simulink model "LeaderFollower"  (R2018a)
settings: Solver=FixedStepAuto  StartTime=0.0  StopTime=300  FixedStep=1  RelTol=1e-3
libraries: simulink x3
settings Model: Creator=wangluo  LastModifiedBy=wangluo

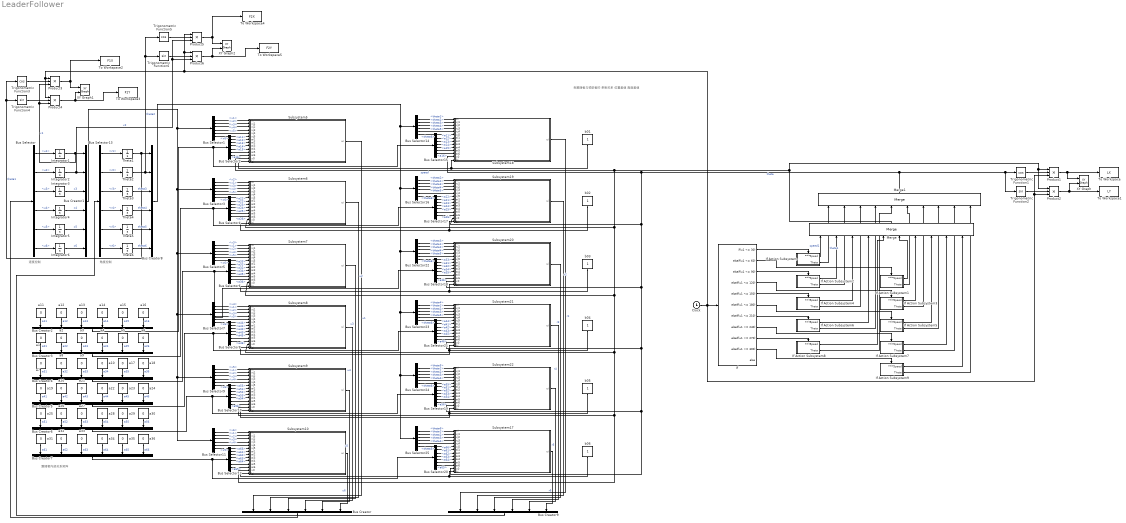
== system LeaderFollower ==
  note: 跟随者内部关系矩阵
  note: 速度控制
  note: 各跟随者与领航者的
      | 牵制关系
      | 位置差值
      | 角度差值
  note: 角度控制
  Bus Creator{,1..9} (10 alike) : BusCreator  Inputs=6
  Bus Selector : BusSelector  OutputSignals=u1,u2,u3,u4,u5,u6
  Bus Selector1 : BusSelector  OutputSignals=x1,x2,x3,x4,x5,x6
  Bus Selector10 : BusSelector  OutputSignals=a55,a51,a52,a53,a54,a56
  Bus Selector11 : BusSelector  OutputSignals=x6,x1,x2,x3,x4,x5
  Bus Selector12 : BusSelector  OutputSignals=a66,a61,a62,a63,a64,a65
  Bus Selector13 : BusSelector  OutputSignals=r1,r2,r3,r4,r5,r6
  Bus Selector14 : BusSelector  OutputSignals=theta1,theta2,theta3,theta4,theta5,theta6
  Bus Selector15 : BusSelector  OutputSignals=a11,a12,a13,a14,a15,a16
  Bus Selector16 : BusSelector  OutputSignals=theta2,theta1,theta3,theta4,theta5,theta6
  Bus Selector17 : BusSelector  OutputSignals=a22,a21,a23,a24,a25,a26
  Bus Selector18 : BusSelector  OutputSignals=a33,a31,a32,a34,a35,a36
  Bus Selector19 : BusSelector  OutputSignals=a55,a51,a52,a53,a54,a56
  Bus Selector2 : BusSelector  OutputSignals=a11,a12,a13,a14,a15,a16
  Bus Selector20 : BusSelector  OutputSignals=a66,a61,a62,a63,a64,a65
  Bus Selector21 : BusSelector  OutputSignals=a44,a41,a42,a43,a45,a46
  Bus Selector22 : BusSelector  OutputSignals=theta3,theta1,theta2,theta4,theta5,theta6
  Bus Selector23 : BusSelector  OutputSignals=theta4,theta1,theta2,theta3,theta5,theta6
  Bus Selector24 : BusSelector  OutputSignals=theta5,theta1,theta2,theta3,theta4,theta6
  Bus Selector25 : BusSelector  OutputSignals=theta6,theta1,theta2,theta3,theta4,theta5
  Bus Selector3 : BusSelector  OutputSignals=x2,x1,x3,x4,x5,x6
  Bus Selector4 : BusSelector  OutputSignals=a22,a21,a23,a24,a25,a26
  Bus Selector5 : BusSelector  OutputSignals=x3,x1,x2,x4,x5,x6
  Bus Selector6 : BusSelector  OutputSignals=a33,a31,a32,a34,a35,a36
  Bus Selector7 : BusSelector  OutputSignals=x4,x1,x2,x3,x5,x6
  Bus Selector8 : BusSelector  OutputSignals=a44,a41,a42,a43,a45,a46
  Bus Selector9 : BusSelector  OutputSignals=x5,x1,x2,x3,x4,x6
  Clock : Clock
      settings: Decimation=280
  If : If  IfExpression=u1 <= 30  ElseIfExpressions=u1 <= 60, u1 <= 90, u1 <= 120, u1 <= 150, u1 <= 180, u1 <= 210, u1 <= 240, u1 <= 270, u1 <= 300
  If Action Subsystem : Subsystem  TreatAsAtomicUnit=on
  If Action Subsystem1 : Subsystem  TreatAsAtomicUnit=on
  If Action Subsystem2 : Subsystem  TreatAsAtomicUnit=on
  If Action Subsystem3 : Subsystem  TreatAsAtomicUnit=on
  If Action Subsystem4 : Subsystem  TreatAsAtomicUnit=on
  If Action Subsystem5 : Subsystem  TreatAsAtomicUnit=on
  If Action Subsystem6 : Subsystem  TreatAsAtomicUnit=on
  If Action Subsystem7 : Subsystem  TreatAsAtomicUnit=on
  If Action Subsystem8 : Subsystem  TreatAsAtomicUnit=on
  If Action Subsystem9 : Subsystem  TreatAsAtomicUnit=on
  Integrator1 : Integrator  InitialCondition=2
  Integrator2 : Integrator  InitialCondition=4
  Integrator3 : Integrator  InitialCondition=6
  Integrator4 : Integrator  InitialCondition=8
  Integrator5 : Integrator  InitialCondition=10
  Integrator6 : Integrator  InitialCondition=2
  Merge : Merge  Inputs=10
  Merge1 : Merge  Inputs=10
  Product{1..6} (6 alike) : Product  Inputs=3
  Subsystem10 : Subsystem
  Subsystem17 : Subsystem
  Subsystem18 : Subsystem
  Subsystem19 : Subsystem
  Subsystem20 : Subsystem
  Subsystem21 : Subsystem
  Subsystem22 : Subsystem
  Subsystem5 : Subsystem
  Subsystem6 : Subsystem
  Subsystem7 : Subsystem
  Subsystem8 : Subsystem
  Subsystem9 : Subsystem
  Theta1 : Integrator
  Theta2 : Integrator  InitialCondition=15
  Theta3 : Integrator  InitialCondition=45
  Theta4 : Integrator  InitialCondition=60
  Theta5 : Integrator  InitialCondition=75
  Theta6 : Integrator  InitialCondition=90
  To Workspace : ToWorkspace  VariableName=LX  SaveFormat=Timeseries  SampleTime=-1
  To Workspace1 : ToWorkspace  VariableName=LY  SaveFormat=Timeseries  SampleTime=-1
  To Workspace2 : ToWorkspace  VariableName=F1X  SaveFormat=Timeseries  SampleTime=-1
  To Workspace3 : ToWorkspace  VariableName=F1Y  SaveFormat=Timeseries  SampleTime=-1
  To Workspace4 : ToWorkspace  VariableName=F2X  SaveFormat=Timeseries  SampleTime=-1
  To Workspace5 : ToWorkspace  VariableName=F2Y  SaveFormat=Timeseries  SampleTime=-1
  Trigonometric Function1 : Trigonometry  Operator=cos
  Trigonometric Function2 : Trigonometry
  Trigonometric Function3 : Trigonometry  Operator=cos
  Trigonometric Function4 : Trigonometry
  Trigonometric Function5 : Trigonometry  Operator=cos
  Trigonometric Function6 : Trigonometry
  XY Graph : simulink/Sinks/XY Graph  xmin=-10  xmax=500  ymin=-10  ymax=500  st=-1
  XY Graph1 : simulink/Sinks/XY Graph  xmin=-10  xmax=500  ymin=-10  ymax=500  st=-1
  XY Graph2 : simulink/Sinks/XY Graph  xmin=-10  xmax=500  ymin=-10  ymax=500  st=-1
  a{1..36} (36 alike) : Constant  Value=0
  b01 : Constant
  b02 : Constant
  b03 : Constant
  b04 : Constant
  b05 : Constant
  b06 : Constant
  wires:
  a8/1 -> Bus Creator4/2  "a32"
  a35/1 -> Bus Creator7/5  "a65"
  Integrator1/1 -> Product4/3, Product3/3, Bus Creator1/1  "x1"
  a19/1 -> Bus Creator5/1  "a41"
  Bus Selector12/1 -> Subsystem10/7(ai1)  "<a66>"
  Bus Selector6/3 -> Subsystem7/9(ai3)  "<a32>"
  Bus Selector9/6 -> Subsystem9/6(xj5)  "<x6>"
  a26/1 -> Bus Creator6/2  "a52"
  Bus Selector4/2 -> Subsystem6/8(ai2)  "<a21>"
  Bus Selector8/1 -> Subsystem8/7(ai1)  "<a44>"
  Integrator3/1 -> Bus Creator1/3  "x3"
  Subsystem8/1(ui) -> Bus Creator/4  "u4"
  Bus Selector10/2 -> Subsystem9/8(ai2)  "<a51>"
  Bus Selector2/4 -> Subsystem5/10(ai4)  "<a14>"
  Bus Selector8/3 -> Subsystem8/9(ai3)  "<a42>"
  Bus Selector12/5 -> Subsystem10/11(ai5)  "<a64>"
  Bus Selector3/5 -> Subsystem6/5(xj4)  "<x5>"
  Bus Selector8/2 -> Subsystem8/8(ai2)  "<a41>"
  a29/1 -> Bus Creator6/5  "a55"
  Bus Selector4/6 -> Subsystem6/12(ai6)  "<a26>"
  Integrator6/1 -> Bus Creator1/6  "x6"
  a23/1 -> Bus Creator5/5  "a45"
  a34/1 -> Bus Creator7/4  "a64"
  Bus Selector3/2 -> Subsystem6/2(xj1)  "<x1>"
  a16/1 -> Bus Creator2/6  "a16"
  a2/1 -> Bus Creator3/2  "a22"
  Bus Selector6/6 -> Subsystem7/12(ai6)  "<a36>"
  Bus Creator4/1 -> Bus Selector18/1, Bus Selector6/1
  Bus Selector2/2 -> Subsystem5/8(ai2)  "<a12>"
  a22/1 -> Bus Creator5/4  "a44"
  Bus Selector7/1 -> Subsystem8/1(xi)  "<x4>"
  Bus Selector7/5 -> Subsystem8/5(xj4)  "<x5>"
  Bus Selector7/2 -> Subsystem8/2(xj1)  "<x1>"
  Bus Creator1/1 -> Bus Selector11/1, Bus Selector9/1, Bus Selector7/1, Bus Selector5/1, Bus Selector3/1, Bus Selector1/1
  Bus Selector1/3 -> Subsystem5/3(xj2)  "<x3>"
  Bus Selector9/3 -> Subsystem9/3(xj2)  "<x2>"
  Bus Selector3/3 -> Subsystem6/3(xj2)  "<x3>"
  a27/1 -> Bus Creator6/3  "a53"
  a31/1 -> Bus Creator7/1  "a61"
  Bus Selector2/5 -> Subsystem5/11(ai5)  "<a15>"
  a15/1 -> Bus Creator2/5  "a15"
  a17/1 -> Bus Creator4/5  "a35"
  Bus Selector9/2 -> Subsystem9/2(xj1)  "<x1>"
  a1/1 -> Bus Creator3/1  "a21"
  Bus Selector12/6 -> Subsystem10/12(ai6)  "<a65>"
  a18/1 -> Bus Creator4/6  "a36"
  a5/1 -> Bus Creator3/5  "a25"
  Bus Selector2/1 -> Subsystem5/7(ai1)  "<a11>"
  Bus Selector4/1 -> Subsystem6/7(ai1)  "<a22>"
  Bus Selector11/4 -> Subsystem10/4(xj3)  "<x3>"
  Bus Selector7/4 -> Subsystem8/4(xj3)  "<x3>"
  Bus Selector12/2 -> Subsystem10/8(ai2)  "<a61>"
  Bus Selector7/3 -> Subsystem8/3(xj2)  "<x2>"
  Bus Selector11/3 -> Subsystem10/3(xj2)  "<x2>"
  a11/1 -> Bus Creator2/1  "a11"
  Bus Creator/1 -> Bus Selector/1
  Bus Selector5/2 -> Subsystem7/2(xj1)  "<x1>"
  Bus Selector2/6 -> Subsystem5/12(ai6)  "<a16>"
  a25/1 -> Bus Creator6/1  "a51"
  Bus Selector1/6 -> Subsystem5/6(xj5)  "<x6>"
  Bus Selector5/6 -> Subsystem7/6(xj5)  "<x6>"
  Bus Selector8/6 -> Subsystem8/12(ai6)  "<a46>"
  Bus Creator7/1 -> Bus Selector20/1, Bus Selector12/1
  Bus Selector5/5 -> Subsystem7/5(xj4)  "<x5>"
  Bus Selector3/1 -> Subsystem6/1(xi)  "<x2>"
  Bus Selector6/4 -> Subsystem7/10(ai4)  "<a34>"
  Bus Selector5/4 -> Subsystem7/4(xj3)  "<x4>"
  a28/1 -> Bus Creator6/4  "a54"
  Bus Selector2/3 -> Subsystem5/9(ai3)  "<a13>"
  Subsystem6/1(ui) -> Bus Creator/2  "u2"
  a13/1 -> Bus Creator2/3  "a13"
  a32/1 -> Bus Creator7/2  "a62"
  Bus Selector1/4 -> Subsystem5/4(xj3)  "<x4>"
  Subsystem5/1(ui) -> Bus Creator/1  "u1"
  Bus Selector10/3 -> Subsystem9/9(ai3)  "<a52>"
  Integrator4/1 -> Bus Creator1/4  "x4"
  Bus Selector5/3 -> Subsystem7/3(xj2)  "<x2>"
  Bus Selector6/2 -> Subsystem7/8(ai2)  "<a31>"
  Bus Selector4/4 -> Subsystem6/10(ai4)  "<a24>"
  Bus Selector11/6 -> Subsystem10/6(xj5)  "<x5>"
  a36/1 -> Bus Creator7/6  "a66"
  Bus Selector4/5 -> Subsystem6/11(ai5)  "<a25>"
  Bus Selector4/3 -> Subsystem6/9(ai3)  "<a23>"
  Bus Selector3/6 -> Subsystem6/6(xj5)  "<x6>"
  Bus Selector5/1 -> Subsystem7/1(xi)  "<x3>"
  Bus Creator6/1 -> Bus Selector19/1, Bus Selector10/1
  Bus Selector7/6 -> Subsystem8/6(xj5)  "<x6>"
  Bus Selector12/4 -> Subsystem10/10(ai4)  "<a63>"
  Bus Selector8/4 -> Subsystem8/10(ai4)  "<a43>"
  Integrator5/1 -> Bus Creator1/5  "x5"
  Bus Selector10/5 -> Subsystem9/11(ai5)  "<a54>"
  Bus Selector1/1 -> Subsystem5/1(xi)  "<x1>"
  Integrator2/1 -> Product6/3, Product5/3, Bus Creator1/2  "x2"
  Bus Selector10/4 -> Subsystem9/10(ai4)  "<a53>"
  Bus Selector8/5 -> Subsystem8/11(ai5)  "<a45>"
  Bus Selector9/1 -> Subsystem9/1(xi)  "<x5>"
  Bus Selector6/1 -> Subsystem7/7(ai1)  "<a33>"
  a33/1 -> Bus Creator7/3  "a63"
  Bus Selector9/4 -> Subsystem9/4(xj3)  "<x3>"
  Subsystem10/1(ui) -> Bus Creator/6  "u6"
  Bus Selector3/4 -> Subsystem6/4(xj3)  "<x4>"
  Bus Creator2/1 -> Bus Selector2/1, Bus Selector15/1
  a21/1 -> Bus Creator5/3  "a43"
  a12/1 -> Bus Creator2/2  "a12"
  a24/1 -> Bus Creator5/6  "a46"
  Bus Selector11/2 -> Subsystem10/2(xj1)  "<x1>"
  Bus Selector6/5 -> Subsystem7/11(ai5)  "<a35>"
  Bus Selector10/6 -> Subsystem9/12(ai6)  "<a56>"
  Bus Selector11/5 -> Subsystem10/5(xj4)  "<x4>"
  Bus Selector9/5 -> Subsystem9/5(xj4)  "<x4>"
  Subsystem7/1(ui) -> Bus Creator/3  "u3"
  a3/1 -> Bus Creator3/3  "a23"
  Bus Selector11/1 -> Subsystem10/1(xi)  "<x6>"
  a20/1 -> Bus Creator5/2  "a42"
  Bus Selector10/1 -> Subsystem9/7(ai1)  "<a55>"
  a6/1 -> Bus Creator3/6  "a26"
  Bus Selector1/5 -> Subsystem5/5(xj4)  "<x5>"
  Bus Selector12/3 -> Subsystem10/9(ai3)  "<a62>"
  a4/1 -> Bus Creator3/4  "a24"
  a10/1 -> Bus Creator4/4  "a34"
  Bus Creator3/1 -> Bus Selector4/1, Bus Selector17/1
  a7/1 -> Bus Creator4/1  "a31"
  Bus Creator5/1 -> Bus Selector8/1, Bus Selector21/1
  a30/1 -> Bus Creator6/6  "a56"
  Bus Selector1/2 -> Subsystem5/2(xj1)  "<x2>"
  a9/1 -> Bus Creator4/3  "a33"
  Subsystem9/1(ui) -> Bus Creator/5  "u5"
  a14/1 -> Bus Creator2/4  "a14"
  Bus Selector/1 -> Integrator1/1  "<u1>"
  Bus Selector/2 -> Integrator2/1  "<u2>"
  Bus Selector/3 -> Integrator3/1  "<u3>"
  Bus Selector/4 -> Integrator4/1  "<u4>"
  Bus Selector/5 -> Integrator5/1  "<u5>"
  Bus Selector/6 -> Integrator6/1  "<u6>"
  Theta1/1 -> Trigonometric Function3/1, Trigonometric Function4/1, Bus Creator8/1  "theta1"
  Theta2/1 -> Trigonometric Function5/1, Trigonometric Function6/1, Bus Creator8/2  "theta2"
  Theta3/1 -> Bus Creator8/3  "theta3"
  Theta5/1 -> Bus Creator8/5  "theta5"
  Theta6/1 -> Bus Creator8/6  "theta6"
  Theta4/1 -> Bus Creator8/4  "theta4"
  Bus Selector13/1 -> Theta1/1  "<r1>"
  Bus Selector13/2 -> Theta2/1  "<r2>"
  Bus Selector13/3 -> Theta3/1  "<r3>"
  Bus Selector13/4 -> Theta4/1  "<r4>"
  Bus Selector13/5 -> Theta5/1  "<r5>"
  Bus Selector13/6 -> Theta6/1  "<r6>"
  Bus Selector14/1 -> Subsystem18/1(xi)  "<theta1>"
  Bus Selector14/2 -> Subsystem18/2(xj1)  "<theta2>"
  Bus Selector14/3 -> Subsystem18/3(xj2)  "<theta3>"
  Bus Selector14/4 -> Subsystem18/4(xj3)  "<theta4>"
  Bus Selector14/5 -> Subsystem18/5(xj4)  "<theta5>"
  Bus Selector14/6 -> Subsystem18/6(xj5)  "<theta6>"
  Bus Creator8/1 -> Bus Selector23/1, Bus Selector25/1, Bus Selector24/1, Bus Selector22/1, Bus Selector16/1, Bus Selector14/1
  Subsystem17/1(ui) -> Bus Creator9/6  "r6"
  Bus Selector15/1 -> Subsystem18/7(ai1)  "<a11>"
  Bus Selector15/2 -> Subsystem18/8(ai2)  "<a12>"
  Bus Selector15/3 -> Subsystem18/9(ai3)  "<a13>"
  Bus Selector15/4 -> Subsystem18/10(ai4)  "<a14>"
  Bus Selector15/5 -> Subsystem18/11(ai5)  "<a15>"
  Bus Selector15/6 -> Subsystem18/12(ai6)  "<a16>"
  Bus Selector17/1 -> Subsystem19/7(ai1)  "<a22>"
  Bus Selector17/2 -> Subsystem19/8(ai2)  "<a21>"
  Bus Selector17/3 -> Subsystem19/9(ai3)  "<a23>"
  Bus Selector17/4 -> Subsystem19/10(ai4)  "<a24>"
  Bus Selector17/5 -> Subsystem19/11(ai5)  "<a25>"
  Bus Selector17/6 -> Subsystem19/12(ai6)  "<a26>"
  Bus Selector16/1 -> Subsystem19/1(xi)  "<theta2>"
  Bus Selector16/2 -> Subsystem19/2(xj1)  "<theta1>"
  Bus Selector16/3 -> Subsystem19/3(xj2)  "<theta3>"
  Bus Selector16/4 -> Subsystem19/4(xj3)  "<theta4>"
  Bus Selector16/5 -> Subsystem19/5(xj4)  "<theta5>"
  Bus Selector16/6 -> Subsystem19/6(xj5)  "<theta6>"
  Bus Selector18/1 -> Subsystem20/7(ai1)  "<a33>"
  Bus Selector18/2 -> Subsystem20/8(ai2)  "<a31>"
  Bus Selector18/3 -> Subsystem20/9(ai3)  "<a32>"
  Bus Selector18/4 -> Subsystem20/10(ai4)  "<a34>"
  Bus Selector18/5 -> Subsystem20/11(ai5)  "<a35>"
  Bus Selector18/6 -> Subsystem20/12(ai6)  "<a36>"
  Bus Selector21/1 -> Subsystem21/7(ai1)  "<a44>"
  Bus Selector21/2 -> Subsystem21/8(ai2)  "<a41>"
  Bus Selector21/3 -> Subsystem21/9(ai3)  "<a42>"
  Bus Selector21/4 -> Subsystem21/10(ai4)  "<a43>"
  Bus Selector21/5 -> Subsystem21/11(ai5)  "<a45>"
  Bus Selector21/6 -> Subsystem21/12(ai6)  "<a46>"
  Bus Selector19/1 -> Subsystem22/7(ai1)  "<a55>"
  Bus Selector19/2 -> Subsystem22/8(ai2)  "<a51>"
  Bus Selector19/3 -> Subsystem22/9(ai3)  "<a52>"
  Bus Selector19/4 -> Subsystem22/10(ai4)  "<a53>"
  Bus Selector19/5 -> Subsystem22/11(ai5)  "<a54>"
  Bus Selector19/6 -> Subsystem22/12(ai6)  "<a56>"
  Bus Selector20/1 -> Subsystem17/7(ai1)  "<a66>"
  Bus Selector20/2 -> Subsystem17/8(ai2)  "<a61>"
  Bus Selector20/3 -> Subsystem17/9(ai3)  "<a62>"
  Bus Selector20/4 -> Subsystem17/10(ai4)  "<a63>"
  Bus Selector20/5 -> Subsystem17/11(ai5)  "<a64>"
  Bus Selector20/6 -> Subsystem17/12(ai6)  "<a65>"
  Subsystem22/1(ui) -> Bus Creator9/5  "r5"
  Subsystem21/1(ui) -> Bus Creator9/4  "r4"
  Subsystem20/1(ui) -> Bus Creator9/3  "r3"
  Subsystem18/1(ui) -> Bus Creator9/1  "r1"
  Subsystem19/1(ui) -> Bus Creator9/2  "r2"
  Bus Creator9/1 -> Bus Selector13/1
  Bus Selector22/1 -> Subsystem20/1(xi)  "<theta3>"
  Bus Selector22/2 -> Subsystem20/2(xj1)  "<theta1>"
  Bus Selector22/3 -> Subsystem20/3(xj2)  "<theta2>"
  Bus Selector22/4 -> Subsystem20/4(xj3)  "<theta4>"
  Bus Selector22/5 -> Subsystem20/5(xj4)  "<theta5>"
  Bus Selector22/6 -> Subsystem20/6(xj5)  "<theta6>"
  Bus Selector23/1 -> Subsystem21/1(xi)  "<theta4>"
  Bus Selector23/2 -> Subsystem21/2(xj1)  "<theta1>"
  Bus Selector23/3 -> Subsystem21/3(xj2)  "<theta2>"
  Bus Selector23/4 -> Subsystem21/4(xj3)  "<theta3>"
  Bus Selector23/5 -> Subsystem21/5(xj4)  "<theta5>"
  Bus Selector23/6 -> Subsystem21/6(xj5)  "<theta6>"
  Bus Selector25/1 -> Subsystem17/1(xi)  "<theta6>"
  Bus Selector25/2 -> Subsystem17/2(xj1)  "<theta1>"
  Bus Selector25/3 -> Subsystem17/3(xj2)  "<theta2>"
  Bus Selector25/4 -> Subsystem17/4(xj3)  "<theta3>"
  Bus Selector25/5 -> Subsystem17/5(xj4)  "<theta4>"
  Bus Selector25/6 -> Subsystem17/6(xj5)  "<theta5>"
  Bus Selector24/1 -> Subsystem22/1(xi)  "<theta5>"
  Bus Selector24/2 -> Subsystem22/2(xj1)  "<theta1>"
  Bus Selector24/3 -> Subsystem22/3(xj2)  "<theta2>"
  Bus Selector24/4 -> Subsystem22/4(xj3)  "<theta3>"
  Bus Selector24/5 -> Subsystem22/5(xj4)  "<theta4>"
  Bus Selector24/6 -> Subsystem22/6(xj5)  "<theta6>"
  b01/1 -> Subsystem18/14(bi), Subsystem5/14(bi)
  b02/1 -> Subsystem19/14(bi), Subsystem6/14(bi)
  b03/1 -> Subsystem20/14(bi), Subsystem7/14(bi)
  b04/1 -> Subsystem8/14(bi), Subsystem21/14(bi)
  b05/1 -> Subsystem9/14(bi), Subsystem22/14(bi)
  b06/1 -> Subsystem17/14(bi), Subsystem10/14(bi)
  Merge1/1 -> Subsystem17/13(x0), Subsystem22/13(x0), Subsystem21/13(x0), Subsystem20/13(x0), Subsystem19/13(x0), Subsystem18/13(x0), Trigonometric Function2/1, Trigonometric Function1/1  "theta"
  Clock/1 -> Product5/1, Product6/1, Product4/1, Product3/1, Product1/3, Product2/3, If/1
  Merge/1 -> Product1/1, Product2/1, Subsystem10/13(x0), Subsystem9/13(x0), Subsystem8/13(x0), Subsystem7/13(x0), Subsystem6/13(x0), Subsystem5/13(x0)  "speed"
  If/1 -> If Action Subsystem/Action
  If/3 -> If Action Subsystem2/Action
  If/5 -> If Action Subsystem4/Action
  If/7 -> If Action Subsystem6/Action
  If/9 -> If Action Subsystem8/Action
  If/2 -> If Action Subsystem1/Action
  If/10 -> If Action Subsystem9/Action
  If/8 -> If Action Subsystem7/Action
  If/6 -> If Action Subsystem5/Action
  If/4 -> If Action Subsystem3/Action
  If Action Subsystem/1(Speed) -> Merge/1  "speed1"
  If Action Subsystem2/1(Speed) -> Merge/2
  If Action Subsystem4/1(Speed) -> Merge/3
  If Action Subsystem6/1(Speed) -> Merge/4
  If Action Subsystem8/1(Speed) -> Merge/5
  If Action Subsystem1/1(Speed) -> Merge/6
  If Action Subsystem3/1(Speed) -> Merge/7
  If Action Subsystem9/1(Speed) -> Merge/10
  If Action Subsystem7/1(Speed) -> Merge/9
  If Action Subsystem5/1(Speed) -> Merge/8
  If Action Subsystem/2(Theta) -> Merge1/1  "theta1"
  If Action Subsystem2/2(Theta) -> Merge1/2
  If Action Subsystem4/2(Theta) -> Merge1/3
  If Action Subsystem6/2(Theta) -> Merge1/4
  If Action Subsystem8/2(Theta) -> Merge1/5
  If Action Subsystem1/2(Theta) -> Merge1/6
  If Action Subsystem3/2(Theta) -> Merge1/7
  If Action Subsystem5/2(Theta) -> Merge1/8
  If Action Subsystem7/2(Theta) -> Merge1/9
  If Action Subsystem9/2(Theta) -> Merge1/10
  Trigonometric Function1/1 -> Product1/2
  Trigonometric Function2/1 -> Product2/2
  Product1/1 -> To Workspace/1, XY Graph/1
  Product2/1 -> To Workspace1/1, XY Graph/2
  Product3/1 -> To Workspace2/1, XY Graph1/1
  Product4/1 -> To Workspace3/1, XY Graph1/2
  Trigonometric Function3/1 -> Product3/2
  Trigonometric Function4/1 -> Product4/2
  Product5/1 -> To Workspace4/1, XY Graph2/1
  Product6/1 -> To Workspace5/1, XY Graph2/2
  Trigonometric Function5/1 -> Product5/2
  Trigonometric Function6/1 -> Product6/2

== system LeaderFollower/If Action Subsystem ==
  Action Port : ActionPort  ActionType=then
  b1 : Constant  Value=5
  b2 : Constant  Value=pi/180*90
  Speed : Outport
  Theta : Outport  Port=2
  wires:
  b1/1 -> Speed/1
  b2/1 -> Theta/1

== system LeaderFollower/If Action Subsystem1 ==
  Action Port : ActionPort  ActionType=elseif
  b1 : Constant  Value=5
  b2 : Constant  Value=pi/180*0
  Speed : Outport
  Theta : Outport  Port=2
  wires:
  b1/1 -> Speed/1
  b2/1 -> Theta/1

== system LeaderFollower/If Action Subsystem2 ==
  Action Port : ActionPort  ActionType=elseif
  b1 : Constant  Value=5
  b2 : Constant  Value=pi/180*45
  Speed : Outport
  Theta : Outport  Port=2
  wires:
  b1/1 -> Speed/1
  b2/1 -> Theta/1

== system LeaderFollower/If Action Subsystem3 ==
  Action Port : ActionPort  ActionType=elseif
  b1 : Constant  Value=5
  b2 : Constant  Value=pi/180*90
  Speed : Outport
  Theta : Outport  Port=2
  wires:
  b1/1 -> Speed/1
  b2/1 -> Theta/1

== system LeaderFollower/If Action Subsystem4 ==
  Action Port : ActionPort  ActionType=elseif
  b1 : Constant  Value=5
  b2 : Constant  Value=pi/180*45
  Speed : Outport
  Theta : Outport  Port=2
  wires:
  b1/1 -> Speed/1
  b2/1 -> Theta/1

== system LeaderFollower/If Action Subsystem5 ==
  Action Port : ActionPort  ActionType=elseif
  b1 : Constant  Value=5
  b2 : Constant  Value=pi/180*0
  Speed : Outport
  Theta : Outport  Port=2
  wires:
  b1/1 -> Speed/1
  b2/1 -> Theta/1

== system LeaderFollower/If Action Subsystem6 ==
  Action Port : ActionPort  ActionType=elseif
  b1 : Constant  Value=5
  b2 : Constant  Value=pi/180*(-45)
  Speed : Outport
  Theta : Outport  Port=2
  wires:
  b1/1 -> Speed/1
  b2/1 -> Theta/1

== system LeaderFollower/If Action Subsystem7 ==
  Action Port : ActionPort  ActionType=elseif
  b1 : Constant  Value=5
  b2 : Constant  Value=pi/180*(-90)
  Speed : Outport
  Theta : Outport  Port=2
  wires:
  b1/1 -> Speed/1
  b2/1 -> Theta/1

== system LeaderFollower/If Action Subsystem8 ==
  Action Port : ActionPort  ActionType=elseif
  b1 : Constant  Value=5
  b2 : Constant  Value=pi/180*(-45)
  Speed : Outport
  Theta : Outport  Port=2
  wires:
  b1/1 -> Speed/1
  b2/1 -> Theta/1

== system LeaderFollower/If Action Subsystem9 ==
  Action Port : ActionPort  ActionType=elseif
  b1 : Constant  Value=5
  b2 : Constant  Value=pi/180*0
  Speed : Outport
  Theta : Outport  Port=2
  wires:
  b1/1 -> Speed/1
  b2/1 -> Theta/1

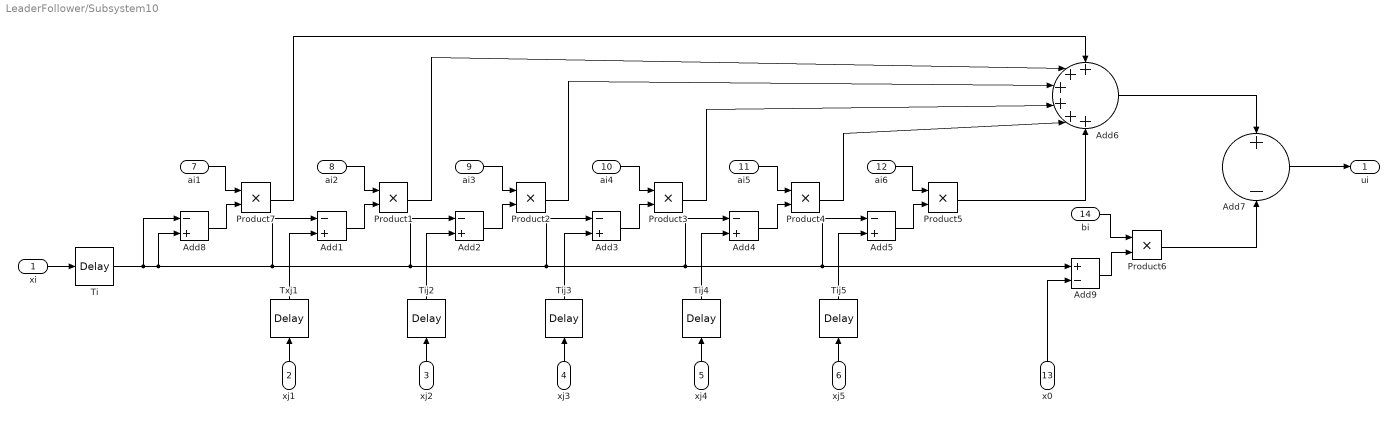
== system LeaderFollower/Subsystem10 ==
  xi : Inport
  xj1 : Inport  Port=2
  xj2 : Inport  Port=3
  xj3 : Inport  Port=4
  xj4 : Inport  Port=5
  xj5 : Inport  Port=6
  ai1 : Inport  Port=7
  ai2 : Inport  Port=8
  ai3 : Inport  Port=9
  ai4 : Inport  Port=10
  ai5 : Inport  Port=11
  ai6 : Inport  Port=12
  x0 : Inport  Port=13
  bi : Inport  Port=14
  Add{1..5,8} (6 alike) : Sum  Inputs=-+
  Add6 : Sum  Inputs=++++++
  Add7 : Sum  Inputs=+-
  Add9 : Sum  Inputs=+-
  Product{1..7} (7 alike) : Product
  Ti : TransportDelay  DelayTime=0
  Tij{2..5} (4 alike) : TransportDelay  DelayTime=0
  Txj1 : TransportDelay  DelayTime=0
  ui : Outport
  wires:
  Product7/1 -> Add6/1
  Add8/1 -> Product7/2
  ai1/1 -> Product7/1
  ai2/1 -> Product1/1
  Add1/1 -> Product1/2
  ai3/1 -> Product2/1
  Add2/1 -> Product2/2
  ai4/1 -> Product3/1
  Add3/1 -> Product3/2
  ai5/1 -> Product4/1
  Add4/1 -> Product4/2
  ai6/1 -> Product5/1
  Add5/1 -> Product5/2
  xi/1 -> Ti/1
  xj5/1 -> Tij5/1
  xj1/1 -> Txj1/1
  Ti/1 -> Add5/1, Add9/1, Add4/1, Add3/1, Add2/1, Add1/1, Add8/2, Add8/1
  Txj1/1 -> Add1/2
  xj2/1 -> Tij2/1
  xj3/1 -> Tij3/1
  xj4/1 -> Tij4/1
  Tij5/1 -> Add5/2
  Tij2/1 -> Add2/2
  Tij3/1 -> Add3/2
  Tij4/1 -> Add4/2
  Product5/1 -> Add6/6
  Product4/1 -> Add6/5
  Product3/1 -> Add6/4
  Product2/1 -> Add6/3
  Product1/1 -> Add6/2
  Add9/1 -> Product6/2
  bi/1 -> Product6/1
  x0/1 -> Add9/2
  Add6/1 -> Add7/1
  Product6/1 -> Add7/2
  Add7/1 -> ui/1

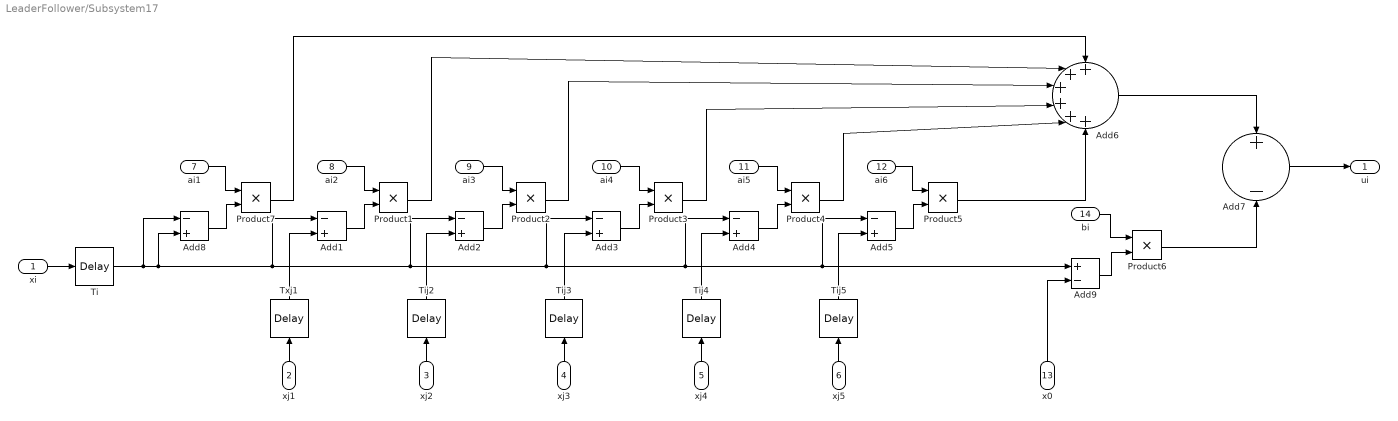
== system LeaderFollower/Subsystem17 ==
  xi : Inport
  xj1 : Inport  Port=2
  xj2 : Inport  Port=3
  xj3 : Inport  Port=4
  xj4 : Inport  Port=5
  xj5 : Inport  Port=6
  ai1 : Inport  Port=7
  ai2 : Inport  Port=8
  ai3 : Inport  Port=9
  ai4 : Inport  Port=10
  ai5 : Inport  Port=11
  ai6 : Inport  Port=12
  x0 : Inport  Port=13
  bi : Inport  Port=14
  Add{1..5,8} (6 alike) : Sum  Inputs=-+
  Add6 : Sum  Inputs=++++++
  Add7 : Sum  Inputs=+-
  Add9 : Sum  Inputs=+-
  Product{1..7} (7 alike) : Product
  Ti : TransportDelay  DelayTime=0
  Tij{2..5} (4 alike) : TransportDelay  DelayTime=0
  Txj1 : TransportDelay  DelayTime=0
  ui : Outport
  wires:
  Product7/1 -> Add6/1
  Add8/1 -> Product7/2
  ai1/1 -> Product7/1
  ai2/1 -> Product1/1
  Add1/1 -> Product1/2
  ai3/1 -> Product2/1
  Add2/1 -> Product2/2
  ai4/1 -> Product3/1
  Add3/1 -> Product3/2
  ai5/1 -> Product4/1
  Add4/1 -> Product4/2
  ai6/1 -> Product5/1
  Add5/1 -> Product5/2
  xi/1 -> Ti/1
  xj5/1 -> Tij5/1
  xj1/1 -> Txj1/1
  Ti/1 -> Add5/1, Add9/1, Add4/1, Add3/1, Add2/1, Add1/1, Add8/2, Add8/1
  Txj1/1 -> Add1/2
  xj2/1 -> Tij2/1
  xj3/1 -> Tij3/1
  xj4/1 -> Tij4/1
  Tij5/1 -> Add5/2
  Tij2/1 -> Add2/2
  Tij3/1 -> Add3/2
  Tij4/1 -> Add4/2
  Product5/1 -> Add6/6
  Product4/1 -> Add6/5
  Product3/1 -> Add6/4
  Product2/1 -> Add6/3
  Product1/1 -> Add6/2
  Add9/1 -> Product6/2
  bi/1 -> Product6/1
  x0/1 -> Add9/2
  Add6/1 -> Add7/1
  Product6/1 -> Add7/2
  Add7/1 -> ui/1

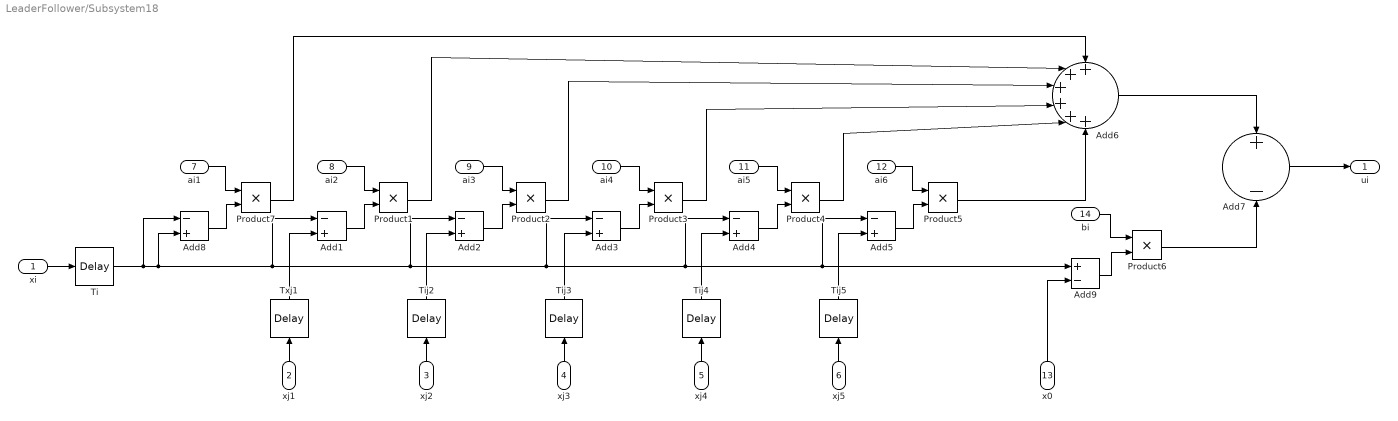
== system LeaderFollower/Subsystem18 ==
  xi : Inport
  xj1 : Inport  Port=2
  xj2 : Inport  Port=3
  xj3 : Inport  Port=4
  xj4 : Inport  Port=5
  xj5 : Inport  Port=6
  ai1 : Inport  Port=7
  ai2 : Inport  Port=8
  ai3 : Inport  Port=9
  ai4 : Inport  Port=10
  ai5 : Inport  Port=11
  ai6 : Inport  Port=12
  x0 : Inport  Port=13
  bi : Inport  Port=14
  Add{1..5,8} (6 alike) : Sum  Inputs=-+
  Add6 : Sum  Inputs=++++++
  Add7 : Sum  Inputs=+-
  Add9 : Sum  Inputs=+-
  Product{1..7} (7 alike) : Product
  Ti : TransportDelay  DelayTime=0
  Tij{2..5} (4 alike) : TransportDelay  DelayTime=0
  Txj1 : TransportDelay  DelayTime=0
  ui : Outport
  wires:
  Product7/1 -> Add6/1
  Add8/1 -> Product7/2
  ai1/1 -> Product7/1
  ai2/1 -> Product1/1
  Add1/1 -> Product1/2
  ai3/1 -> Product2/1
  Add2/1 -> Product2/2
  ai4/1 -> Product3/1
  Add3/1 -> Product3/2
  ai5/1 -> Product4/1
  Add4/1 -> Product4/2
  ai6/1 -> Product5/1
  Add5/1 -> Product5/2
  xi/1 -> Ti/1
  xj5/1 -> Tij5/1
  xj1/1 -> Txj1/1
  Ti/1 -> Add5/1, Add9/1, Add4/1, Add3/1, Add2/1, Add1/1, Add8/2, Add8/1
  Txj1/1 -> Add1/2
  xj2/1 -> Tij2/1
  xj3/1 -> Tij3/1
  xj4/1 -> Tij4/1
  Tij5/1 -> Add5/2
  Tij2/1 -> Add2/2
  Tij3/1 -> Add3/2
  Tij4/1 -> Add4/2
  Product5/1 -> Add6/6
  Product4/1 -> Add6/5
  Product3/1 -> Add6/4
  Product2/1 -> Add6/3
  Product1/1 -> Add6/2
  Add9/1 -> Product6/2
  bi/1 -> Product6/1
  x0/1 -> Add9/2
  Add6/1 -> Add7/1
  Product6/1 -> Add7/2
  Add7/1 -> ui/1

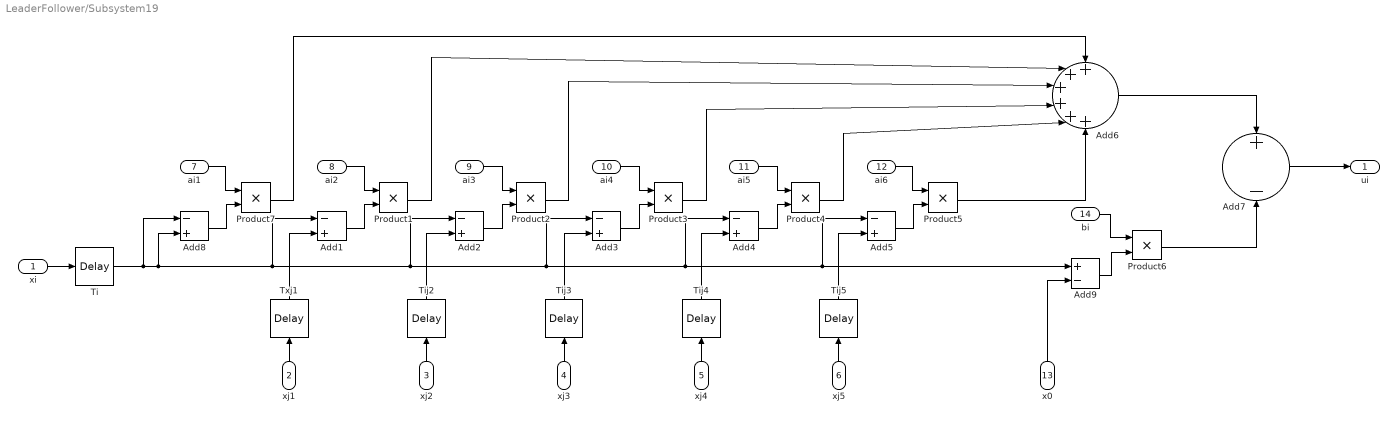
== system LeaderFollower/Subsystem19 ==
  xi : Inport
  xj1 : Inport  Port=2
  xj2 : Inport  Port=3
  xj3 : Inport  Port=4
  xj4 : Inport  Port=5
  xj5 : Inport  Port=6
  ai1 : Inport  Port=7
  ai2 : Inport  Port=8
  ai3 : Inport  Port=9
  ai4 : Inport  Port=10
  ai5 : Inport  Port=11
  ai6 : Inport  Port=12
  x0 : Inport  Port=13
  bi : Inport  Port=14
  Add{1..5,8} (6 alike) : Sum  Inputs=-+
  Add6 : Sum  Inputs=++++++
  Add7 : Sum  Inputs=+-
  Add9 : Sum  Inputs=+-
  Product{1..7} (7 alike) : Product
  Ti : TransportDelay  DelayTime=0
  Tij{2..5} (4 alike) : TransportDelay  DelayTime=0
  Txj1 : TransportDelay  DelayTime=0
  ui : Outport
  wires:
  Product7/1 -> Add6/1
  Add8/1 -> Product7/2
  ai1/1 -> Product7/1
  ai2/1 -> Product1/1
  Add1/1 -> Product1/2
  ai3/1 -> Product2/1
  Add2/1 -> Product2/2
  ai4/1 -> Product3/1
  Add3/1 -> Product3/2
  ai5/1 -> Product4/1
  Add4/1 -> Product4/2
  ai6/1 -> Product5/1
  Add5/1 -> Product5/2
  xi/1 -> Ti/1
  xj5/1 -> Tij5/1
  xj1/1 -> Txj1/1
  Ti/1 -> Add5/1, Add9/1, Add4/1, Add3/1, Add2/1, Add1/1, Add8/2, Add8/1
  Txj1/1 -> Add1/2
  xj2/1 -> Tij2/1
  xj3/1 -> Tij3/1
  xj4/1 -> Tij4/1
  Tij5/1 -> Add5/2
  Tij2/1 -> Add2/2
  Tij3/1 -> Add3/2
  Tij4/1 -> Add4/2
  Product5/1 -> Add6/6
  Product4/1 -> Add6/5
  Product3/1 -> Add6/4
  Product2/1 -> Add6/3
  Product1/1 -> Add6/2
  Add9/1 -> Product6/2
  bi/1 -> Product6/1
  x0/1 -> Add9/2
  Add6/1 -> Add7/1
  Product6/1 -> Add7/2
  Add7/1 -> ui/1

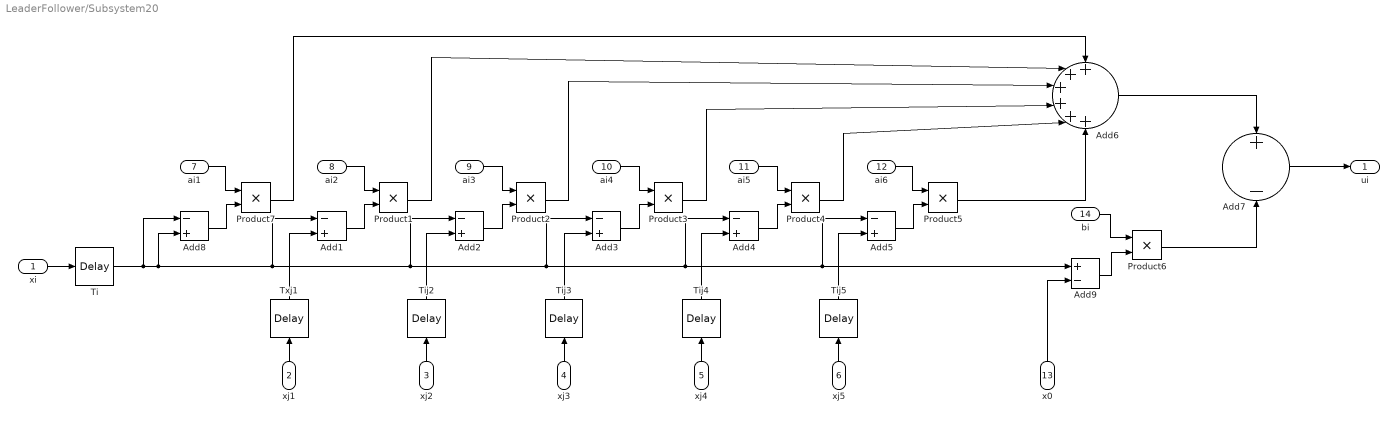
== system LeaderFollower/Subsystem20 ==
  xi : Inport
  xj1 : Inport  Port=2
  xj2 : Inport  Port=3
  xj3 : Inport  Port=4
  xj4 : Inport  Port=5
  xj5 : Inport  Port=6
  ai1 : Inport  Port=7
  ai2 : Inport  Port=8
  ai3 : Inport  Port=9
  ai4 : Inport  Port=10
  ai5 : Inport  Port=11
  ai6 : Inport  Port=12
  x0 : Inport  Port=13
  bi : Inport  Port=14
  Add{1..5,8} (6 alike) : Sum  Inputs=-+
  Add6 : Sum  Inputs=++++++
  Add7 : Sum  Inputs=+-
  Add9 : Sum  Inputs=+-
  Product{1..7} (7 alike) : Product
  Ti : TransportDelay  DelayTime=0
  Tij{2..5} (4 alike) : TransportDelay  DelayTime=0
  Txj1 : TransportDelay  DelayTime=0
  ui : Outport
  wires:
  Product7/1 -> Add6/1
  Add8/1 -> Product7/2
  ai1/1 -> Product7/1
  ai2/1 -> Product1/1
  Add1/1 -> Product1/2
  ai3/1 -> Product2/1
  Add2/1 -> Product2/2
  ai4/1 -> Product3/1
  Add3/1 -> Product3/2
  ai5/1 -> Product4/1
  Add4/1 -> Product4/2
  ai6/1 -> Product5/1
  Add5/1 -> Product5/2
  xi/1 -> Ti/1
  xj5/1 -> Tij5/1
  xj1/1 -> Txj1/1
  Ti/1 -> Add5/1, Add9/1, Add4/1, Add3/1, Add2/1, Add1/1, Add8/2, Add8/1
  Txj1/1 -> Add1/2
  xj2/1 -> Tij2/1
  xj3/1 -> Tij3/1
  xj4/1 -> Tij4/1
  Tij5/1 -> Add5/2
  Tij2/1 -> Add2/2
  Tij3/1 -> Add3/2
  Tij4/1 -> Add4/2
  Product5/1 -> Add6/6
  Product4/1 -> Add6/5
  Product3/1 -> Add6/4
  Product2/1 -> Add6/3
  Product1/1 -> Add6/2
  Add9/1 -> Product6/2
  bi/1 -> Product6/1
  x0/1 -> Add9/2
  Add6/1 -> Add7/1
  Product6/1 -> Add7/2
  Add7/1 -> ui/1

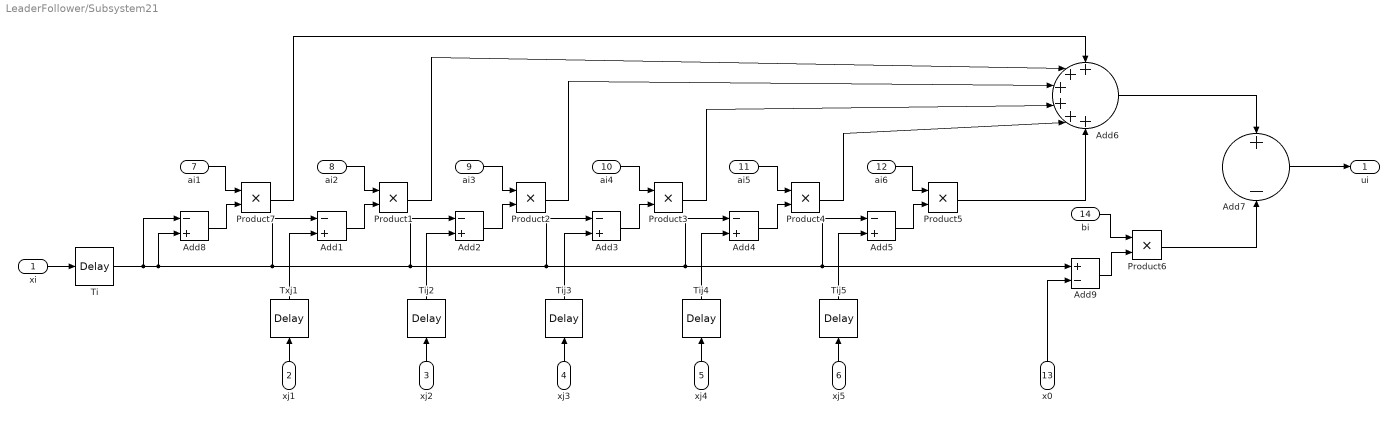
== system LeaderFollower/Subsystem21 ==
  xi : Inport
  xj1 : Inport  Port=2
  xj2 : Inport  Port=3
  xj3 : Inport  Port=4
  xj4 : Inport  Port=5
  xj5 : Inport  Port=6
  ai1 : Inport  Port=7
  ai2 : Inport  Port=8
  ai3 : Inport  Port=9
  ai4 : Inport  Port=10
  ai5 : Inport  Port=11
  ai6 : Inport  Port=12
  x0 : Inport  Port=13
  bi : Inport  Port=14
  Add{1..5,8} (6 alike) : Sum  Inputs=-+
  Add6 : Sum  Inputs=++++++
  Add7 : Sum  Inputs=+-
  Add9 : Sum  Inputs=+-
  Product{1..7} (7 alike) : Product
  Ti : TransportDelay  DelayTime=0
  Tij{2..5} (4 alike) : TransportDelay  DelayTime=0
  Txj1 : TransportDelay  DelayTime=0
  ui : Outport
  wires:
  Product7/1 -> Add6/1
  Add8/1 -> Product7/2
  ai1/1 -> Product7/1
  ai2/1 -> Product1/1
  Add1/1 -> Product1/2
  ai3/1 -> Product2/1
  Add2/1 -> Product2/2
  ai4/1 -> Product3/1
  Add3/1 -> Product3/2
  ai5/1 -> Product4/1
  Add4/1 -> Product4/2
  ai6/1 -> Product5/1
  Add5/1 -> Product5/2
  xi/1 -> Ti/1
  xj5/1 -> Tij5/1
  xj1/1 -> Txj1/1
  Ti/1 -> Add5/1, Add9/1, Add4/1, Add3/1, Add2/1, Add1/1, Add8/2, Add8/1
  Txj1/1 -> Add1/2
  xj2/1 -> Tij2/1
  xj3/1 -> Tij3/1
  xj4/1 -> Tij4/1
  Tij5/1 -> Add5/2
  Tij2/1 -> Add2/2
  Tij3/1 -> Add3/2
  Tij4/1 -> Add4/2
  Product5/1 -> Add6/6
  Product4/1 -> Add6/5
  Product3/1 -> Add6/4
  Product2/1 -> Add6/3
  Product1/1 -> Add6/2
  Add9/1 -> Product6/2
  bi/1 -> Product6/1
  x0/1 -> Add9/2
  Add6/1 -> Add7/1
  Product6/1 -> Add7/2
  Add7/1 -> ui/1

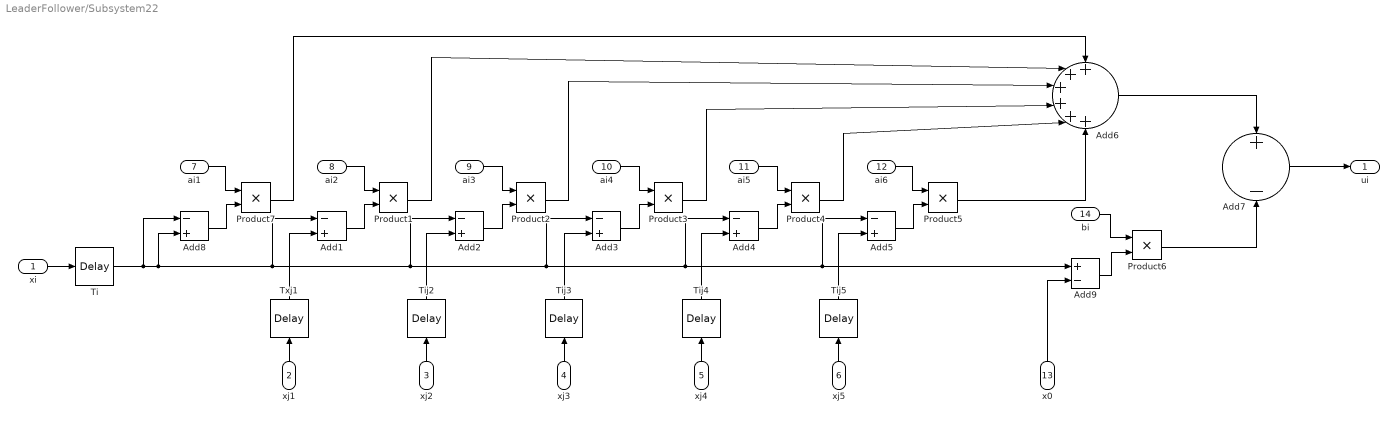
== system LeaderFollower/Subsystem22 ==
  xi : Inport
  xj1 : Inport  Port=2
  xj2 : Inport  Port=3
  xj3 : Inport  Port=4
  xj4 : Inport  Port=5
  xj5 : Inport  Port=6
  ai1 : Inport  Port=7
  ai2 : Inport  Port=8
  ai3 : Inport  Port=9
  ai4 : Inport  Port=10
  ai5 : Inport  Port=11
  ai6 : Inport  Port=12
  x0 : Inport  Port=13
  bi : Inport  Port=14
  Add{1..5,8} (6 alike) : Sum  Inputs=-+
  Add6 : Sum  Inputs=++++++
  Add7 : Sum  Inputs=+-
  Add9 : Sum  Inputs=+-
  Product{1..7} (7 alike) : Product
  Ti : TransportDelay  DelayTime=0
  Tij{2..5} (4 alike) : TransportDelay  DelayTime=0
  Txj1 : TransportDelay  DelayTime=0
  ui : Outport
  wires:
  Product7/1 -> Add6/1
  Add8/1 -> Product7/2
  ai1/1 -> Product7/1
  ai2/1 -> Product1/1
  Add1/1 -> Product1/2
  ai3/1 -> Product2/1
  Add2/1 -> Product2/2
  ai4/1 -> Product3/1
  Add3/1 -> Product3/2
  ai5/1 -> Product4/1
  Add4/1 -> Product4/2
  ai6/1 -> Product5/1
  Add5/1 -> Product5/2
  xi/1 -> Ti/1
  xj5/1 -> Tij5/1
  xj1/1 -> Txj1/1
  Ti/1 -> Add5/1, Add9/1, Add4/1, Add3/1, Add2/1, Add1/1, Add8/2, Add8/1
  Txj1/1 -> Add1/2
  xj2/1 -> Tij2/1
  xj3/1 -> Tij3/1
  xj4/1 -> Tij4/1
  Tij5/1 -> Add5/2
  Tij2/1 -> Add2/2
  Tij3/1 -> Add3/2
  Tij4/1 -> Add4/2
  Product5/1 -> Add6/6
  Product4/1 -> Add6/5
  Product3/1 -> Add6/4
  Product2/1 -> Add6/3
  Product1/1 -> Add6/2
  Add9/1 -> Product6/2
  bi/1 -> Product6/1
  x0/1 -> Add9/2
  Add6/1 -> Add7/1
  Product6/1 -> Add7/2
  Add7/1 -> ui/1

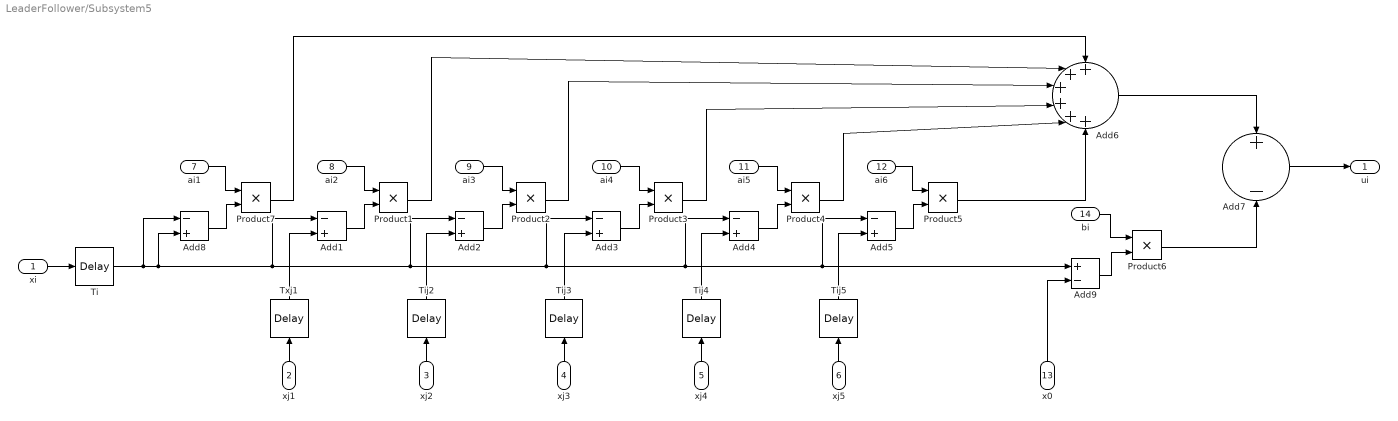
== system LeaderFollower/Subsystem5 ==
  xi : Inport
  xj1 : Inport  Port=2
  xj2 : Inport  Port=3
  xj3 : Inport  Port=4
  xj4 : Inport  Port=5
  xj5 : Inport  Port=6
  ai1 : Inport  Port=7
  ai2 : Inport  Port=8
  ai3 : Inport  Port=9
  ai4 : Inport  Port=10
  ai5 : Inport  Port=11
  ai6 : Inport  Port=12
  x0 : Inport  Port=13
  bi : Inport  Port=14
  Add{1..5,8} (6 alike) : Sum  Inputs=-+
  Add6 : Sum  Inputs=++++++
  Add7 : Sum  Inputs=+-
  Add9 : Sum  Inputs=+-
  Product{1..7} (7 alike) : Product
  Ti : TransportDelay  DelayTime=0
  Tij{2..5} (4 alike) : TransportDelay  DelayTime=0
  Txj1 : TransportDelay  DelayTime=0
  ui : Outport
  wires:
  Product7/1 -> Add6/1
  Add8/1 -> Product7/2
  ai1/1 -> Product7/1
  ai2/1 -> Product1/1
  Add1/1 -> Product1/2
  ai3/1 -> Product2/1
  Add2/1 -> Product2/2
  ai4/1 -> Product3/1
  Add3/1 -> Product3/2
  ai5/1 -> Product4/1
  Add4/1 -> Product4/2
  ai6/1 -> Product5/1
  Add5/1 -> Product5/2
  xi/1 -> Ti/1
  xj5/1 -> Tij5/1
  xj1/1 -> Txj1/1
  Ti/1 -> Add5/1, Add9/1, Add4/1, Add3/1, Add2/1, Add1/1, Add8/2, Add8/1
  Txj1/1 -> Add1/2
  xj2/1 -> Tij2/1
  xj3/1 -> Tij3/1
  xj4/1 -> Tij4/1
  Tij5/1 -> Add5/2
  Tij2/1 -> Add2/2
  Tij3/1 -> Add3/2
  Tij4/1 -> Add4/2
  Product5/1 -> Add6/6
  Product4/1 -> Add6/5
  Product3/1 -> Add6/4
  Product2/1 -> Add6/3
  Product1/1 -> Add6/2
  Add9/1 -> Product6/2
  bi/1 -> Product6/1
  x0/1 -> Add9/2
  Add6/1 -> Add7/1
  Product6/1 -> Add7/2
  Add7/1 -> ui/1

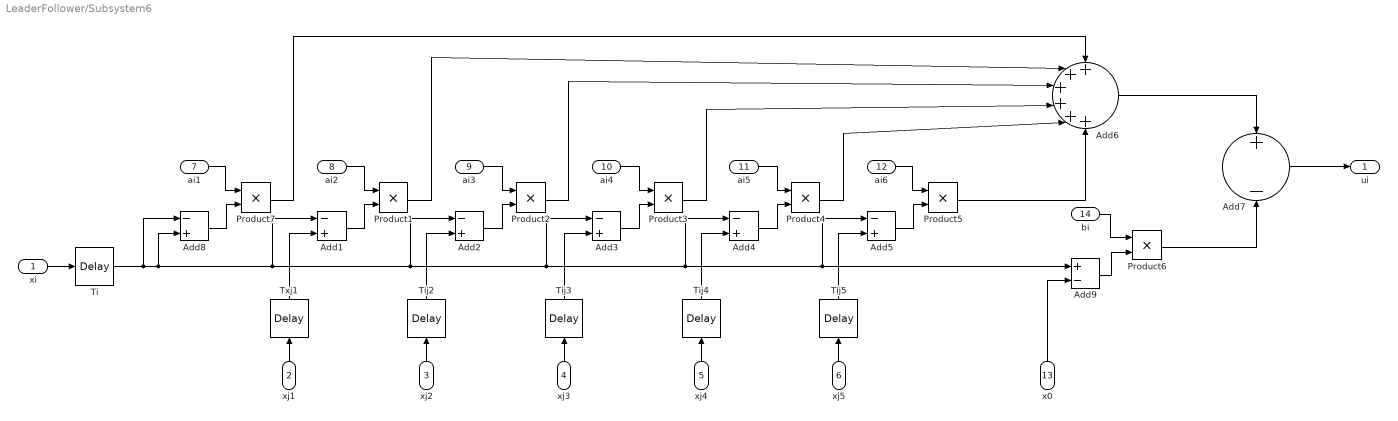
== system LeaderFollower/Subsystem6 ==
  xi : Inport
  xj1 : Inport  Port=2
  xj2 : Inport  Port=3
  xj3 : Inport  Port=4
  xj4 : Inport  Port=5
  xj5 : Inport  Port=6
  ai1 : Inport  Port=7
  ai2 : Inport  Port=8
  ai3 : Inport  Port=9
  ai4 : Inport  Port=10
  ai5 : Inport  Port=11
  ai6 : Inport  Port=12
  x0 : Inport  Port=13
  bi : Inport  Port=14
  Add{1..5,8} (6 alike) : Sum  Inputs=-+
  Add6 : Sum  Inputs=++++++
  Add7 : Sum  Inputs=+-
  Add9 : Sum  Inputs=+-
  Product{1..7} (7 alike) : Product
  Ti : TransportDelay  DelayTime=0
  Tij{2..5} (4 alike) : TransportDelay  DelayTime=0
  Txj1 : TransportDelay  DelayTime=0
  ui : Outport
  wires:
  Product7/1 -> Add6/1
  Add8/1 -> Product7/2
  ai1/1 -> Product7/1
  ai2/1 -> Product1/1
  Add1/1 -> Product1/2
  ai3/1 -> Product2/1
  Add2/1 -> Product2/2
  ai4/1 -> Product3/1
  Add3/1 -> Product3/2
  ai5/1 -> Product4/1
  Add4/1 -> Product4/2
  ai6/1 -> Product5/1
  Add5/1 -> Product5/2
  xi/1 -> Ti/1
  xj5/1 -> Tij5/1
  xj1/1 -> Txj1/1
  Ti/1 -> Add5/1, Add9/1, Add4/1, Add3/1, Add2/1, Add1/1, Add8/2, Add8/1
  Txj1/1 -> Add1/2
  xj2/1 -> Tij2/1
  xj3/1 -> Tij3/1
  xj4/1 -> Tij4/1
  Tij5/1 -> Add5/2
  Tij2/1 -> Add2/2
  Tij3/1 -> Add3/2
  Tij4/1 -> Add4/2
  Product5/1 -> Add6/6
  Product4/1 -> Add6/5
  Product3/1 -> Add6/4
  Product2/1 -> Add6/3
  Product1/1 -> Add6/2
  Add9/1 -> Product6/2
  bi/1 -> Product6/1
  x0/1 -> Add9/2
  Add6/1 -> Add7/1
  Product6/1 -> Add7/2
  Add7/1 -> ui/1

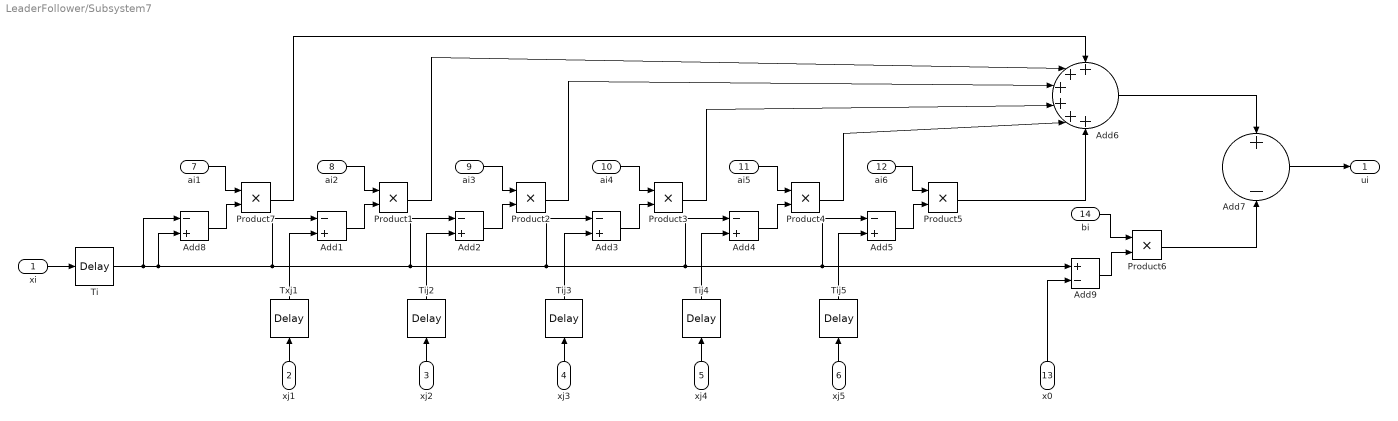
== system LeaderFollower/Subsystem7 ==
  xi : Inport
  xj1 : Inport  Port=2
  xj2 : Inport  Port=3
  xj3 : Inport  Port=4
  xj4 : Inport  Port=5
  xj5 : Inport  Port=6
  ai1 : Inport  Port=7
  ai2 : Inport  Port=8
  ai3 : Inport  Port=9
  ai4 : Inport  Port=10
  ai5 : Inport  Port=11
  ai6 : Inport  Port=12
  x0 : Inport  Port=13
  bi : Inport  Port=14
  Add{1..5,8} (6 alike) : Sum  Inputs=-+
  Add6 : Sum  Inputs=++++++
  Add7 : Sum  Inputs=+-
  Add9 : Sum  Inputs=+-
  Product{1..7} (7 alike) : Product
  Ti : TransportDelay  DelayTime=0
  Tij{2..5} (4 alike) : TransportDelay  DelayTime=0
  Txj1 : TransportDelay  DelayTime=0
  ui : Outport
  wires:
  Product7/1 -> Add6/1
  Add8/1 -> Product7/2
  ai1/1 -> Product7/1
  ai2/1 -> Product1/1
  Add1/1 -> Product1/2
  ai3/1 -> Product2/1
  Add2/1 -> Product2/2
  ai4/1 -> Product3/1
  Add3/1 -> Product3/2
  ai5/1 -> Product4/1
  Add4/1 -> Product4/2
  ai6/1 -> Product5/1
  Add5/1 -> Product5/2
  xi/1 -> Ti/1
  xj5/1 -> Tij5/1
  xj1/1 -> Txj1/1
  Ti/1 -> Add5/1, Add9/1, Add4/1, Add3/1, Add2/1, Add1/1, Add8/2, Add8/1
  Txj1/1 -> Add1/2
  xj2/1 -> Tij2/1
  xj3/1 -> Tij3/1
  xj4/1 -> Tij4/1
  Tij5/1 -> Add5/2
  Tij2/1 -> Add2/2
  Tij3/1 -> Add3/2
  Tij4/1 -> Add4/2
  Product5/1 -> Add6/6
  Product4/1 -> Add6/5
  Product3/1 -> Add6/4
  Product2/1 -> Add6/3
  Product1/1 -> Add6/2
  Add9/1 -> Product6/2
  bi/1 -> Product6/1
  x0/1 -> Add9/2
  Add6/1 -> Add7/1
  Product6/1 -> Add7/2
  Add7/1 -> ui/1

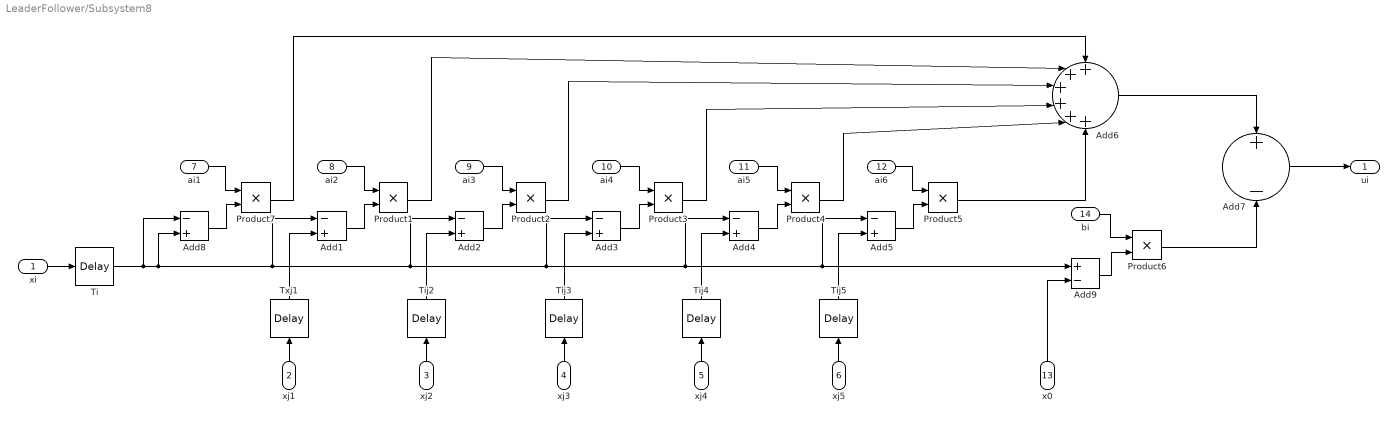
== system LeaderFollower/Subsystem8 ==
  xi : Inport
  xj1 : Inport  Port=2
  xj2 : Inport  Port=3
  xj3 : Inport  Port=4
  xj4 : Inport  Port=5
  xj5 : Inport  Port=6
  ai1 : Inport  Port=7
  ai2 : Inport  Port=8
  ai3 : Inport  Port=9
  ai4 : Inport  Port=10
  ai5 : Inport  Port=11
  ai6 : Inport  Port=12
  x0 : Inport  Port=13
  bi : Inport  Port=14
  Add{1..5,8} (6 alike) : Sum  Inputs=-+
  Add6 : Sum  Inputs=++++++
  Add7 : Sum  Inputs=+-
  Add9 : Sum  Inputs=+-
  Product{1..7} (7 alike) : Product
  Ti : TransportDelay  DelayTime=0
  Tij{2..5} (4 alike) : TransportDelay  DelayTime=0
  Txj1 : TransportDelay  DelayTime=0
  ui : Outport
  wires:
  Product7/1 -> Add6/1
  Add8/1 -> Product7/2
  ai1/1 -> Product7/1
  ai2/1 -> Product1/1
  Add1/1 -> Product1/2
  ai3/1 -> Product2/1
  Add2/1 -> Product2/2
  ai4/1 -> Product3/1
  Add3/1 -> Product3/2
  ai5/1 -> Product4/1
  Add4/1 -> Product4/2
  ai6/1 -> Product5/1
  Add5/1 -> Product5/2
  xi/1 -> Ti/1
  xj5/1 -> Tij5/1
  xj1/1 -> Txj1/1
  Ti/1 -> Add5/1, Add9/1, Add4/1, Add3/1, Add2/1, Add1/1, Add8/2, Add8/1
  Txj1/1 -> Add1/2
  xj2/1 -> Tij2/1
  xj3/1 -> Tij3/1
  xj4/1 -> Tij4/1
  Tij5/1 -> Add5/2
  Tij2/1 -> Add2/2
  Tij3/1 -> Add3/2
  Tij4/1 -> Add4/2
  Product5/1 -> Add6/6
  Product4/1 -> Add6/5
  Product3/1 -> Add6/4
  Product2/1 -> Add6/3
  Product1/1 -> Add6/2
  Add9/1 -> Product6/2
  bi/1 -> Product6/1
  x0/1 -> Add9/2
  Add6/1 -> Add7/1
  Product6/1 -> Add7/2
  Add7/1 -> ui/1

== system LeaderFollower/Subsystem9 ==
  xi : Inport
  xj1 : Inport  Port=2
  xj2 : Inport  Port=3
  xj3 : Inport  Port=4
  xj4 : Inport  Port=5
  xj5 : Inport  Port=6
  ai1 : Inport  Port=7
  ai2 : Inport  Port=8
  ai3 : Inport  Port=9
  ai4 : Inport  Port=10
  ai5 : Inport  Port=11
  ai6 : Inport  Port=12
  x0 : Inport  Port=13
  bi : Inport  Port=14
  Add{1..5,8} (6 alike) : Sum  Inputs=-+
  Add6 : Sum  Inputs=++++++
  Add7 : Sum  Inputs=+-
  Add9 : Sum  Inputs=+-
  Product{1..7} (7 alike) : Product
  Ti : TransportDelay  DelayTime=0
  Tij{2..5} (4 alike) : TransportDelay  DelayTime=0
  Txj1 : TransportDelay  DelayTime=0
  ui : Outport
  wires:
  Product7/1 -> Add6/1
  Add8/1 -> Product7/2
  ai1/1 -> Product7/1
  ai2/1 -> Product1/1
  Add1/1 -> Product1/2
  ai3/1 -> Product2/1
  Add2/1 -> Product2/2
  ai4/1 -> Product3/1
  Add3/1 -> Product3/2
  ai5/1 -> Product4/1
  Add4/1 -> Product4/2
  ai6/1 -> Product5/1
  Add5/1 -> Product5/2
  xi/1 -> Ti/1
  xj5/1 -> Tij5/1
  xj1/1 -> Txj1/1
  Ti/1 -> Add5/1, Add9/1, Add4/1, Add3/1, Add2/1, Add1/1, Add8/2, Add8/1
  Txj1/1 -> Add1/2
  xj2/1 -> Tij2/1
  xj3/1 -> Tij3/1
  xj4/1 -> Tij4/1
  Tij5/1 -> Add5/2
  Tij2/1 -> Add2/2
  Tij3/1 -> Add3/2
  Tij4/1 -> Add4/2
  Product5/1 -> Add6/6
  Product4/1 -> Add6/5
  Product3/1 -> Add6/4
  Product2/1 -> Add6/3
  Product1/1 -> Add6/2
  Add9/1 -> Product6/2
  bi/1 -> Product6/1
  x0/1 -> Add9/2
  Add6/1 -> Add7/1
  Product6/1 -> Add7/2
  Add7/1 -> ui/1
